simulink library "mech_friction"  (Simulink 7.1)
PostLoadFcn:
  | find_system(gcs,'FollowLinks', 'on', 'LookUnderMasks', 'all');
libraries: mblibv1 x6
Description:
  | Static and Kinetic Friction Library
  | 
  | This demo library contains blocks that allow you to actuate a single joint primitive at a time with these types of friction:
  | 
  | * A mix of static and kinetic contact friction, proportional to static and kinetic friction coefficients and the force normal to the contact surface
  | * Kinetic damping friction proportional to joint primitive velocity, either translational or rotational, but with opposite sign
  | 
  | These demo library blocks are masked subsystems containing SimMechanics and Simulink blocks.
  | 
  | The mixed static-kinetic friction block makes use of the Joint Stiction Actuator block from the SimMechanics Sensors & Actuators Library.  If the connected joint primitive locks, that degree of freedom (DoF) is removed from the system.  SimMechanics tests for locking and unlocking conditions with algebraic loops (non-time-based simulation steps) that can decrease the accuracy of your simulation, particularly if you use a fixed-step solver.  Use such Joint Stiction Actuator blocks only if you need to lock and unlock jonits.
  | 
  | The kinetic damping friction block is a force element that applies a continuous friction force or torque via joint actuation using joint motion measured by a joint sensor.
settings Model: Creator=arnav  LastModifiedBy=batserve

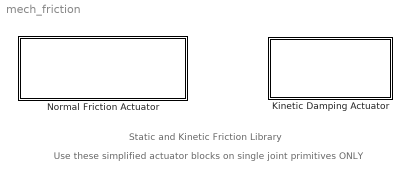
== system mech_friction ==
  note: Static and Kinetic Friction Library
  note: Use these simplified actuator blocks on single joint primitives ONLY
  Kinetic Damping Actuator : Subsystem  mask(Kinetic Damping Actuator){dampingCoeff=0.75, dForce=off, primitive=P1}
      mask prompts: dampingCoeff "Kinetic damping coefficient"; dForce "Show kinetic damping force port"; primitive "Joint primitive"
      mask help:
      | Applies kinetic damping friction to a joint primitive. The friction force/torque is proportional to the velocity of the joint primitive and opposed to its motion. The damping coefficient mu should be positive. The applied friction force/torque is -mu*(joint primitive velocity).
      |
      | Connect the round mechanical connection port to an actuator port on the Joint. You can friction actuate a prismatic or revolute primitive, but not a spherical primitive.
      |
      | The joint primitive menu lists all possible primitives. You must select the correct primitive after you connect the actuator to the joint.
      mask init:
      | %mech_kineticDampingActuator(gcb,'setPrimitive');
      | mech_kineticDampingActuator(gcb,'showHideFrictionForces',dForce);
      settings: CopyFcn=|
      | %set_param(gcb,'LinkStatus','none');
      | %set_param(gcb,'CopyFcn','');
      mask StyleString: edit,checkbox,popup(P1|P2|P3|R1|R2|R3)
  Normal Friction Actuator : Subsystem  AncestorBlock=mech_friction/Normal Friction Actuator  mask(Normal Friction Actuator){Ckinetic=0.05, staticFF=1.55, Csforward=0.055, Csreverse=0.055, sExtActuation=off, sForces=off, primitive=P1}
      mask prompts: Ckinetic "Kinetic friction coefficient"; staticFF "Static friction coefficient"; Csforward "Forward stiction coefficient"; Csreverse "Reverse stiction coefficient"; sExtActuation "Show external actuation port"; sForces "Show kinetic and static friction ports"; primitive "Joint primitive"
      mask help:
      | Applies kinetic and static contact friction to a joint primitive. The friction force/torque is proportional to the force normal to the frictional surfaces in contact. In order for the actuated joint to be able to lock, the static friction coefficient muS must be larger than the kinetic friction coefficient muK. The friction force is mu*(normal force). The coefficient mu should be positive.
      |
      | Connect the round mechanical connection port to an actuator port on the Joint. You can friction actuate a prismatic or revolute primitive, but not a spherical primitive.
      |
      | The joint primitive menu lists all possible primitives. You must select the correct primitive after you connect the actuator to the joint.
      mask init:
      | Csforward = staticFF*Ckinetic;
      | Csreverse = staticFF*Ckinetic;
      | mech_normalFrictionActuator(gcb,'setPrimitive');
      | mech_normalFrictionActuator(gcb,'showHideActuatorSignal',sExtActuation);
      | mech_normalFrictionActuator(gcb,'showHideFrictionForces',sForces);
      settings: CopyFcn=|
      | %set_param(gcb,'LinkStatus','none');
      | %set_param(gcb,'CopyFcn','');
      mask StyleString: edit,edit,edit,edit,checkbox,checkbox,popup(P1|P2|P3|R1|R2|R3)
      mask CallbackString: ||||||%populateStictionPrimitiveList(gcb);

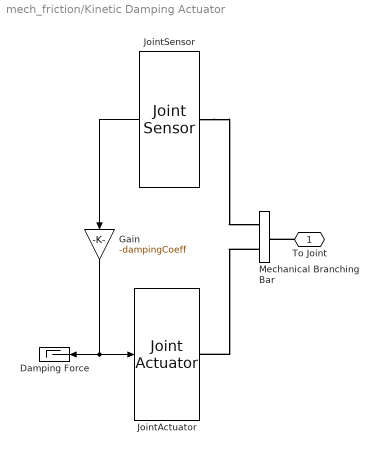
== system mech_friction/Kinetic Damping Actuator ==
  Damping Force : Terminator
  Gain : Gain  Orientation=down  Gain=-dampingCoeff  ParameterDataType=sfix(16)  ParameterScaling=2^0  OutDataType=sfix(16)  OutScaling=2^0
  JointActuator : mblibv1/Sensors &  Actuators/Joint Actuator  DialogController=MECH.DynMechDlgSource  SystemSampleTime=-1  PhysicalDomain=Mechanical  PortType=blob  ActuationStyle=Force  AngleUnits=deg  ArcVelocityUnits=deg/s  ArcAccelerationUnits=deg/s^2  CoordPositionUnits=m  VelocityUnits=m/s  AccelerationUnits=m/s^2  ForceUnits=N  TorqueUnits=N-m  ActiveIO=off  Width=1  DialogClass=MechanicalActuatorBlock  Primitive=P1  ReferenceFrame=Absolute (INERTIAL)
  JointSensor : mblibv1/Sensors &  Actuators/Joint Sensor  Orientation=left  DialogController=MECH.DynMechDlgSource  SystemSampleTime=-1  PhysicalDomain=Mechanical  PortType=blob  Muxed=off  Pose=off  Angle=off  AngleUnits=deg  ArcVelocity=on  ArcVelocityUnits=rad/s  ArcAcceleration=off  ArcAccelerationUnits=deg/s^2  CoordPosition=off  CoordPositionUnits=m  Velocity=on  VelocityUnits=m/s  Acceleration=off  AccelerationUnits=m/s^2  Quaternion=on  QuaternionDT=off  QuaternionDDT=off  QuaternionUnits=deg  OutputVector=[ 1 ]  ActiveIO=off  Width=5  DialogClass=MechanicalSensorBlock  Primitive=P1  Force=off  ForceUnits=N  Torque=off  TorqueUnits=N-m  ReferenceFrame=Absolute (INERTIAL)  ReactionSensedSide=Base  ReactionReferenceFrame=Absolute (World)  ReactionForce=off  ReactionForceUnits=N  ReactionMoment=off  ReactionMomentUnits=N-m
  Mechanical Branching Bar : mblibv1/Utilities/Mechanical Branching Bar  Orientation=left  DialogController=MECH.DynMechDlgSource  PhysicalDomain=mechanical  SubClassName=Unknown  LeftPortType=blob  RightPortType=blob  LConnTagsString=_newl0  RConnTagsString=SA0|SA1  DialogClass=MechanicalBranchingBarBlock  NumSAPorts=2
  To Joint : PMIOPort  Orientation=left  Port=1  Side=Left
  wires:
  JointSensor/1 -> Gain/1
  Gain/1 -> Damping Force/1, JointActuator/1
  connections:
  To Joint/RConn1 -- Mechanical Branching Bar/LConn1
  JointSensor/LConn1 -- Mechanical Branching Bar/RConn1
  Mechanical Branching Bar/RConn2 -- JointActuator/RConn1

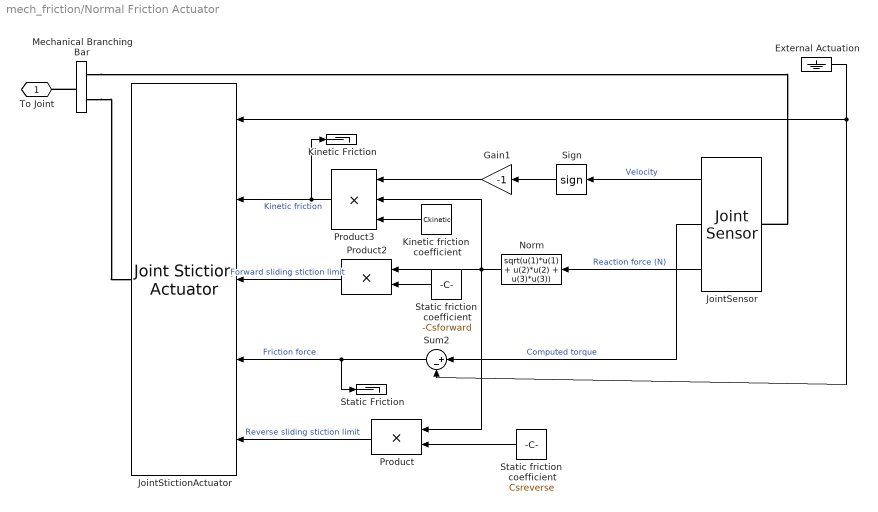
== system mech_friction/Normal Friction Actuator ==
  External Actuation : Ground
  Gain1 : Gain  Orientation=left  Gain=-1  ParameterDataType=sfix(16)  ParameterScaling=2^0  OutDataType=sfix(16)  OutScaling=2^0  SaturateOnIntegerOverflow=on  OutDataTypeStr=Inherit: Same as input  ParamDataTypeStr=Inherit: Same as input
  JointSensor : mblibv1/Sensors &  Actuators/Joint Sensor  Orientation=left  DialogController=MECH.DynMechDlgSource  SystemSampleTime=-1  PhysicalDomain=Mechanical  PortType=blob  Muxed=off  Pose=off  Angle=off  AngleUnits=deg  ArcVelocity=on  ArcVelocityUnits=rad/s  ArcAcceleration=off  ArcAccelerationUnits=deg/s^2  CoordPosition=off  CoordPositionUnits=m  Velocity=on  VelocityUnits=m/s  Acceleration=off  AccelerationUnits=m/s^2  Quaternion=on  QuaternionDT=off  QuaternionDDT=off  QuaternionUnits=deg  OutputVector=[ 1 1 3 ]  ActiveIO=off  Width=5  DialogClass=MechanicalSensorBlock  Primitive=P1  Force=on  ForceUnits=N  Torque=on  TorqueUnits=N-m  ReferenceFrame=Absolute (INERTIAL)  ReactionSensedSide=Base  ReactionReferenceFrame=Absolute (World)  ReactionForce=on  ReactionForceUnits=N  ReactionMoment=off  ReactionMomentUnits=N-m
  JointStictionActuator : mblibv1/Sensors &  Actuators/Joint Stiction Actuator  Orientation=left  DialogController=MECH.DynMechDlgSource  SystemSampleTime=-1  PhysicalDomain=Mechanical  PortType=blob  ActuationStyle=Force  AngleUnits=deg  ArcVelocityUnits=deg/s  ArcAccelerationUnits=deg/s^2  CoordPositionUnits=m  VelocityUnits=m/s  AccelerationUnits=m/s^2  ForceUnits=N  TorqueUnits=N-m  ActiveIO=off  Width=5  DialogClass=EventActuatorBlock  Primitive=P1  FrictionalForceUnits=N  ExternalForceUnits=N  FrictionalTorqueUnits=N-m  ExternalTorqueUnits=N-m  LockingTolerance=1e-2
  Kinetic Friction : Terminator
  Kinetic friction  coefficient : Constant  Orientation=left  Value=Ckinetic  OutDataType=sfix(16)  OutScaling=2^0
  Mechanical Branching Bar : mblibv1/Utilities/Mechanical Branching Bar  DialogController=MECH.DynMechDlgSource  PhysicalDomain=mechanical  SubClassName=Unknown  LeftPortType=blob  RightPortType=blob  LConnTagsString=_newl0  RConnTagsString=SA0|SA1  DialogClass=MechanicalBranchingBarBlock  NumSAPorts=2
  Norm : Fcn  Orientation=left  Expr=sqrt(u(1)*u(1) + u(2)*u(2) + u(3)*u(3))
  Product : Product  Orientation=left  OutDataType=sfix(16)  OutScaling=2^0  SaturateOnIntegerOverflow=on  InputSameDT=on  OutDataTypeStr=Inherit: Same as first input
  Product2 : Product  Orientation=left  OutDataType=sfix(16)  OutScaling=2^0  SaturateOnIntegerOverflow=on  InputSameDT=on  OutDataTypeStr=Inherit: Same as first input
  Product3 : Product  Orientation=left  Inputs=3  OutDataType=sfix(16)  OutScaling=2^0  SaturateOnIntegerOverflow=on  InputSameDT=on  OutDataTypeStr=Inherit: Same as first input
  Sign : Signum  Orientation=left  ZeroCross=off
  Static Friction : Terminator
  Static friction  coefficient : Constant  Orientation=left  Value=Csreverse  OutDataType=sfix(16)  OutScaling=2^0
  "Static friction  coefficient " : Constant  Orientation=left  Value=-Csforward  OutDataType=sfix(16)  OutScaling=2^0
  Sum2 : Sum  Orientation=left  Inputs=|+-  OutDataType=sfix(16)  OutScaling=2^0  SaturateOnIntegerOverflow=on  InputSameDT=on  OutDataTypeStr=Inherit: Same as first input
  To Joint : PMIOPort  Port=1  Side=Left
  wires:
  "Static friction  coefficient "/1 -> Product2/2
  External Actuation/1 -> Sum2/2, JointStictionActuator/1
  Sum2/1 -> Static Friction/1, JointStictionActuator/4  "Friction force"
  JointSensor/2 -> Sum2/1  "Computed torque"
  Static friction  coefficient/1 -> Product/2
  Product3/1 -> Kinetic Friction/1, JointStictionActuator/2  "Kinetic friction"
  Kinetic friction  coefficient/1 -> Product3/3
  Gain1/1 -> Product3/1
  Norm/1 -> Product/1, Product2/1, Product3/2
  Product2/1 -> JointStictionActuator/3  "Forward sliding stiction limit"
  Product/1 -> JointStictionActuator/5  "Reverse sliding stiction limit"
  JointSensor/3 -> Norm/1  "Reaction force (N)"
  Sign/1 -> Gain1/1
  JointSensor/1 -> Sign/1  "Velocity"
  connections:
  Mechanical Branching Bar/RConn1 -- JointSensor/LConn1
  Mechanical Branching Bar/LConn1 -- To Joint/RConn1
  Mechanical Branching Bar/RConn2 -- JointStictionActuator/RConn1
